simulink model "PWMControllerDCMotor_V2"  (R2023b)
settings: Solver=VariableStepAuto  StartTime=0.0  StopTime=25  RelTol=1e-3
values from neighbouring files (symbols this model uses):
  m_resistance = 1.20677778    [LQRJoe.m]    (also in LQRScript.m)
  motor_b = 0.29352    [LQRJoe.m]    (also in LQRScript.m)
  motor_j = 0.0327    [LQRJoe.m]    (also in LQRScript.m)
undefined symbols (not defined in the file or in its folder): m_inductance, m_kb, m_kt
libraries: SignalEditorBlockLib x1
settings Model: Creator=user  LastModifiedBy=user

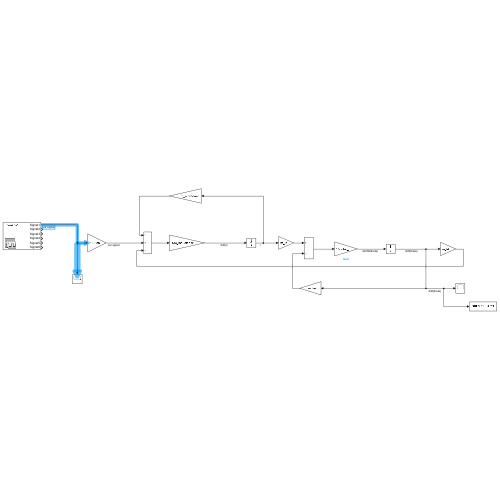
[thumbnail: Simulink's stored preview of the top-level diagram]
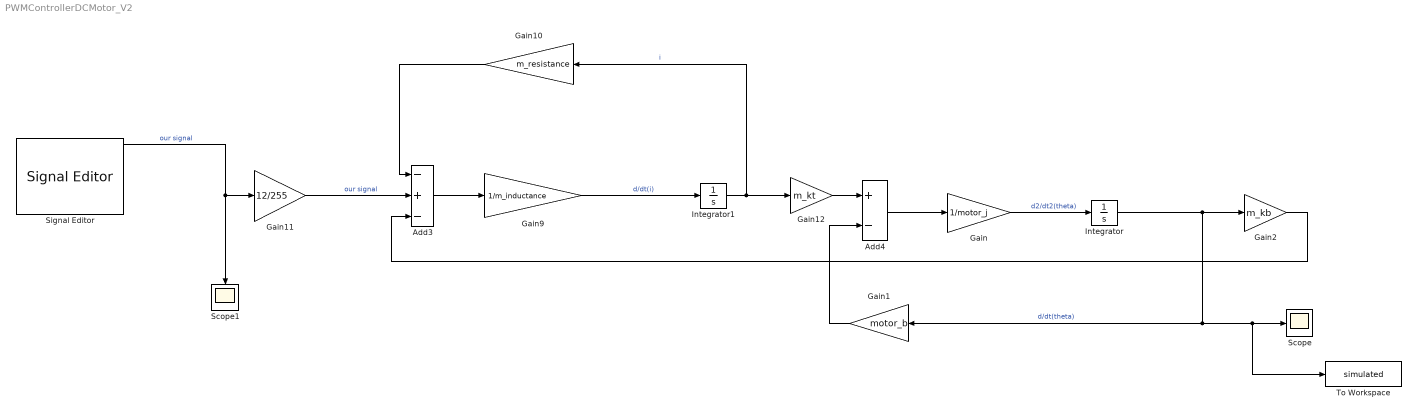
== system PWMControllerDCMotor_V2 ==
  Add3 : Sum  Inputs=-+-
  Add4 : Sum  Inputs=+-
  Gain : Gain  Gain=1/motor_j
  Gain1 : Gain  Gain=motor_b
  Gain10 : Gain  Gain=m_resistance
  Gain11 : Gain  Gain=12/255
  Gain12 : Gain  Gain=m_kt
  Gain2 : Gain  Gain=m_kb
  Gain9 : Gain  Gain=1/m_inductance
  Integrator : Integrator
  Integrator1 : Integrator
  Scope : Scope
  Scope1 : Scope
  Signal Editor : SignalEditorBlockLib/Signal Editor  FileName=MySignals.mat  ActiveScenario=Scenario1  ActiveSignal=Signal1  IsBus=off  OutputBusObjectStr=Bus: BusObject  SampleTime=0  Interpolate=off  ZeroCross=off  OutputAfterFinalValue=Setting to zero  Unit=inherit  PreserveSignalName=on  ApplySigPropsToAllScenarios=on  ApplySigPropsToAllSignals=off
  To Workspace : ToWorkspace  VariableName=simulated  SaveFormat=Timeseries  SampleTime=-1
  wires:
  Gain12/1 -> Add4/1
  Signal Editor/1 -> Scope1/1, Gain11/1  "our signal"
  Gain11/1 -> Add3/2  "our signal"
  Gain9/1 -> Integrator1/1  "d/dt(i)"
  Add3/1 -> Gain9/1
  Gain10/1 -> Add3/1
  Integrator1/1 -> Gain12/1, Gain10/1  "i"
  Add4/1 -> Gain/1
  Gain/1 -> Integrator/1  "d2/dt2(theta)"
  Integrator/1 -> Gain2/1, To Workspace/1, Scope/1, Gain1/1  "d/dt(theta)"
  Gain1/1 -> Add4/2
  Gain2/1 -> Add3/3
